simulink model "sim1"  (R2023b)
settings: Solver=FixedStepAuto  StartTime=0.0  StopTime=0.1  FixedStep=dt  RelTol=1e-3
undefined symbols (not defined in the file): C, dt, L, R
settings Model: Creator=user  LastModifiedBy=witold

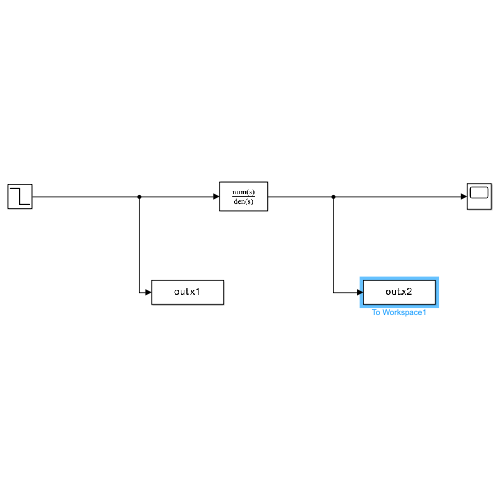
[thumbnail: Simulink's stored preview of the top-level diagram]
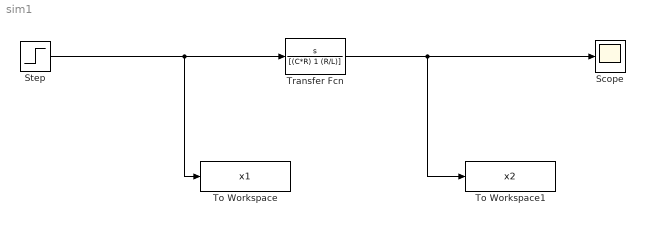
== system sim1 ==
  Scope : Scope
  Step : Step  Time=dt  Before=1  After=0  SampleTime=0
  To Workspace : ToWorkspace  VariableName=x1  SampleTime=-1
  To Workspace1 : ToWorkspace  VariableName=x2  SampleTime=-1
  Transfer Fcn : TransferFcn  Numerator=[1 0]  Denominator=[(C*R) 1 (R/L)]
  wires:
  Step/1 -> To Workspace/1, Transfer Fcn/1
  Transfer Fcn/1 -> To Workspace1/1, Scope/1
